simulink model "BMS_V4"  (R2017b)
settings: Solver=FixedStepDiscrete  StartTime=0.0  StopTime=inf  FixedStep=BASETIME  RelTol=1e-3  EnableMultiTasking=on
values from neighbouring files (symbols this model uses):
  AKT_BALANCE = uint16(8)    [BMS_V4_config.m]
  BALANCE = uint16(4)    [BMS_V4_config.m]
  BALANCE_RESISTOR = int32(5)    [BMS_V4_config.m]
  BALANCE_VEC = uint16(8)    [BMS_V4_config.m]
  CELL_SOC = uint16(7)    [BMS_V4_config.m]
  CELL_STATE = uint16(3)    [BMS_V4_config.m]
  CELL_TEMPERATURE = uint16(6)    [BMS_V4_config.m]
  CELL_VOLTAGE = uint16(5)    [BMS_V4_config.m]
  CELLACTBITFIELD = hex2dec('300')    [BMS_V4_config.m]
  CELLDEACTBITFIELD = hex2dec('100')    [BMS_V4_config.m]
  CELLT_BURST = uint16(6)    [BMS_V4_config.m]
  CELLV_BURST = uint16(5)    [BMS_V4_config.m]
  CLK_CYC_timer_1 = 586    [BMS_V4_config.m]
  CLK_CYC_timer_2 = 5860    [BMS_V4_config.m]
  CLK_CYC_timer_3 = 280    [BMS_V4_config.m]
  CLK_CYC_timer_4 = 586*100    (= 58600)    [BMS_V4_config.m]
  CLK_CYC_timer_5 = 5800*2    (= 11600)    [BMS_V4_config.m]
  CLK_CYC_timer_6 = 320    [BMS_V4_config.m]
  CN_CELLS = int32(40*3600)    [BMS_V4_config.m]
  CONTACTOR = uint16(1)    [BMS_V4_config.m]
  CONTACTOR_LOCKED = uint16(0)    [BMS_V4_config.m]
  CONTACTOR_UNLOCKED = uint16(1)    [BMS_V4_config.m]
  DEBUG_SEND_STATES = uint16(hex2dec('01'))    [BMS_V4_config.m]
  DELTA_SOC_BALANCE = int32(5*1e6)    [BMS_V4_config.m]
  DELTA_SOC_BALANCE_OFF = int32(1*1e5)    [BMS_V4_config.m]
  DETERMINE_MODEL_PARAMETER_ACT = uint16(100)    [BMS_V4_config.m]
  DETERMINE_MODEL_PARAMETER_SCC = uint16(101)    [BMS_V4_config.m]
  ERROR = uint16(1)    [BMS_V4_config.m]
  EXTERN_SIGNALS = uint16(1)    [BMS_V4_config.m]
  FREQUENCY_STEPS = uint16([25 50 75 100 150 250 500 750                                      1000 1500 2500 5000 7500                                      10010 10015 10025 10050 10075                                      10100 10150 10250 10500 10750                                      11000 11500])    [BMS_V4_config.m]
  GET_IMAG_PART_MFC = uint16(9)    [BMS_V4_config.m]
  GET_IMAG_PART_MSF = uint16(4)    [BMS_V4_config.m]
  GET_REAL_PART_MFC = uint16(8)    [BMS_V4_config.m]
  GET_REAL_PART_MSF = uint16(3)    [BMS_V4_config.m]
  IMU = uint16(7)    [BMS_V4_config.m]
  IMU_AMP_OFF = uint16(5)    [BMS_V4_config.m]
  IMU_DATA_READ_LOCUS_ACT = uint16(6)    [BMS_V4_config.m]
  IMU_DATA_READ_LOCUS_SCC = uint16(7)    [BMS_V4_config.m]
  IMU_DEBUG = uint16(9)    [BMS_V4_config.m]
  IMU_GET_DATA_MFC = uint16(8)    [BMS_V4_config.m]
  IMU_GET_DATA_MSF = uint16(3)    [BMS_V4_config.m]
  IMU_OFFSET_POLLING = uint16(11)    [BMS_V4_config.m]
  IMU_POLLING = uint16(2)    [BMS_V4_config.m]
  IMU_POWER = uint16(10)    [BMS_V4_config.m]
  IMU_SEND_IMAG = uint16(11)    [BMS_V4_config.m]
  IMU_SEND_REAL = uint16(10)    [BMS_V4_config.m]
  INDEX_IMAGPART = uint16(2)    [BMS_V4_config.m]
  INDEX_REALPART = uint16(1)    [BMS_V4_config.m]
  INFO = uint16(2)    [BMS_V4_config.m]
  INIT_OFFSET_AMPLITUDE = uint16(2)    [BMS_V4_config.m]
  LINE_CURRENT = uint16(3)    [BMS_V4_config.m]
  LINE_CURRENT_CANA = uint16(4)    [BMS_V4_config.m]
  LINE_CURRENT_SWITCH_THRESHOLD = int32(2*1e6)    [BMS_V4_config.m]
  NUM_OF_CELLS = uint16(16)    [BMS_V4_config.m]
  NUM_OF_FREQUENCIES_PSO = uint16(14)    [BMS_V4_config.m]
  NUM_OF_LINES = uint16(1)    [BMS_V4_config.m]
  NUM_OF_PARAMETER = single(5)    [BMS_V4_config.m]
  NUM_OF_SOC_POINTS = uint16(110)    [BMS_V4_config.m]
  P_L_BOUND = single([0.05;0.01;0.1;0.01;0.1])    [BMS_V4_config.m]
  P_U_BOUND = single([0.50;0.20;0.9;0.06;60])    [BMS_V4_config.m]
  PARA_ACT_SEND = uint16(101)    [BMS_V4_config.m]
  PARA_DATA_STORE_ACT = uint16(8)    [BMS_V4_config.m]
  PARA_DATA_STORE_SCC = uint16(9)    [BMS_V4_config.m]
  PARA_SCC_SEND = uint16(102)    [BMS_V4_config.m]
  PARTICLE_INIT = single(create_startparticle(P_L_BOUND,P_U_BOUND,NUM_OF_PARTICLE))    [BMS_V4_config.m]
  POLACT = hex2dec('00000BFF')    [BMS_V4_config.m]
  POLDEACT = hex2dec('000008FF')    [BMS_V4_config.m]
  PSO_PARA_DEBUG = uint16(13)    [BMS_V4_config.m]
  REQUEST_SOC_REF = uint16(1000)    [BMS_V4_config.m]
  SCALE_FACTOR_CH1 = single(0.66666666)    [BMS_V4_config.m]
  SCALE_FACTOR_CH2 = single(0.66666666)    [BMS_V4_config.m]
  SEND_CELL_SOC_ABS = uint16(199)    [BMS_V4_config.m]
  SHUT_DOWN_BALANCE_OFF = uint16(3)    [BMS_V4_config.m]
  SHUT_DOWN_BALANCE_ON = uint16(2)    [BMS_V4_config.m]
  START_IMU_MSL = uint16(3)    [BMS_V4_config.m]
  START_IMU_SCC = uint16(1)    [BMS_V4_config.m]
  SWITCH_IMU_OFF = uint16(2)    [BMS_V4_config.m]
  SWITCH_IMU_ON = uint16(1)    [BMS_V4_config.m]
  SWITCH_IMU_ON_OFF = uint16(4)    [BMS_V4_config.m]
  SYSTEM_DEBUG = uint16(12)    [BMS_V4_config.m]
  TIMEOUT_CANA = uint32(5000)    [BMS_V4_config.m]
  TIMEOUT_GATEWAY = uint32(500)    [BMS_V4_config.m]
  TS_SOC = single(0.010)    [BMS_V4_config.m]
  WARNING = uint16(2)    [BMS_V4_config.m]
libraries: c280xlib x44, c2833xlib x5, simulink x2, c2000lib x1, idelinklib_common x1
(part 7 of 8)

== matlab function BMS_V4/FunctionCall_CANA_RX/handle_imu_debug/proceeding_imu_debug ==
  data: msg input; imu_function data_store_memory; imu_offset data_store_memory; imu_amplitude data_store_memory; START_IMU_MSL parameter; START_IMU_SCC parameter; INIT_OFFSET_AMPLITUDE parameter; user_imu_request data_store_memory; SWITCH_IMU_ON_OFF parameter; imu_CAN_high data_store_memory; imu_CAN_low data_store_memory; SWITCH_IMU_ON parameter; SWITCH_IMU_OFF parameter; imu_on_off data_store_memory; IMU_POWER parameter; IMU parameter; gateway_request data_store_memory
function imu_debug(msg,START_IMU_MSL,START_IMU_SCC,...
    INIT_OFFSET_AMPLITUDE,SWITCH_IMU_ON_OFF, SWITCH_IMU_ON,...
    SWITCH_IMU_OFF, IMU_POWER,IMU)

global imu_function
global imu_offset;
global imu_amplitude;
global user_imu_request;
global imu_CAN_high;
global imu_CAN_low;
global imu_on_off;
global gateway_request;

x1 = uint16(bitand(uint32(hex2dec('000000FF')),bitshift(msg(1),-0)));

if x1 == uint16(START_IMU_SCC)
    %imu_function=START_IMU_SCC;
    user_imu_request=START_IMU_SCC;

    elseif x1 == uint16(INIT_OFFSET_AMPLITUDE) % Offset und Amplitude. 
         imu_offset = uint16(bitand(uint32(hex2dec('0000FFFF')),...
              bitshift(msg(1),-8)));
         imu_amplitude = uint16(bitor(bitand(uint32(hex2dec('000000FF')),...
              bitshift(msg(1),-24)),bitand(uint32(hex2dec('0000FF00')),...
              bitshift(msg(2),8))));
                       
    elseif x1 == START_IMU_MSL %start manual impedance measurement
        user_imu_request=START_IMU_MSL;
        
    elseif x1 == SWITCH_IMU_ON_OFF %start manual impedance measurement
        on_off = uint16(bitand(uint32(hex2dec('000000FF')),bitshift(msg(1),-8)));
        CODE = uint16([IMU_POWER 0 0 0]);
        imu_CAN_high = uint32(0);
        if on_off == SWITCH_IMU_ON %IMU on
           CODE(2) = SWITCH_IMU_ON; %IMU ON  
           imu_on_off = true;
        else
           CODE(2) = SWITCH_IMU_OFF; %IMU OFF   
           imu_on_off = false;

        end
        x1=uint16(bitand(uint16(hex2dec('00ff')),uint16(CODE(1))));
        x2=uint16(bitand(uint16(hex2dec('ff00')),uint16(bitshift(uint16(CODE(2)),8))));
        x3=uint16(bitand(uint16(hex2dec('00ff')),uint16(CODE(3))));
        x4=uint16(bitand(uint16(hex2dec('ff00')),uint16(bitshift(uint16(CODE(4)),8))));
        x11=uint16(bitor(x1,x2));
        x12=uint16(bitor(x3,x4));
        imu_CAN_low=uint32(bitor(uint32(x11),bitshift(uint32(x12),16)));
        gateway_request(IMU) = true;


        
   

else
    
end
end

== matlab function BMS_V4/FunctionCall_timer_2/calculation_soc_CC ==
  data: cell_voltages data_store_memory; TS_SOC parameter; NUM_OF_CELLS parameter; BALANCE_RESISTOR parameter; cell_soc_ABS data_store_memory; cell_soc_CC data_store_memory; CN_CELLS parameter; line_currents data_store_memory; imu_offset_is_set data_store_memory; imu_offset data_store_memory; balance_vector data_store_memory; imu_cc_scc data_store_memory; imu_function data_store_memory; START_IMU_SCC parameter
function calculation_soc_CC(TS_SOC, NUM_OF_CELLS, BALANCE_RESISTOR,CN_CELLS,START_IMU_SCC)

global imu_offset_is_set;
global imu_offset;
global cell_voltages;
global line_currents;
global balance_vector;
global cell_soc_CC;  %SoC cells coulomb counting
global cell_soc_ABS;
global imu_cc_scc;
global imu_function;


% IMU_offset Offsetcurrent in mA!

%dt=TS_SOC*ones(NUM_OF_CELLS,1);

linoNo = uint16(1);

if imu_offset_is_set == true
   Iges=single(...
        (single(balance_vector).* ... % I balance in mA
        (single(cell_voltages)./(single(1e4)*... %voltage in V
        single(BALANCE_RESISTOR))).*single(-1))+... 
        (single(line_currents(linoNo))/single(1e6)));       % line current to A
        Iges=Iges-(single(imu_offset)/single(1e3));
  
else
   Iges=single(...
        (single(balance_vector).* ... % I balance in mA
        (single(cell_voltages)./(single(1e4)*... %voltage in V
        single(BALANCE_RESISTOR))).*single(-1))+... 
        (single(line_currents(linoNo))/single(1e6)));       % line current to A
end
 
if (imu_function == START_IMU_SCC)
    if imu_offset_is_set == true
        Iges_scc = single(line_currents(linoNo))/single(1e6);
        Iges_scc = Iges_scc-(single(imu_offset)/single(1e3));
    else
        Iges_scc = single(line_currents(linoNo))/single(1e6);
    end
    delta_SoC_scc =  int32(((TS_SOC*Iges_scc)/single(CN_CELLS))*1e8);
else
    delta_SoC_scc =  int32(0);
end

Iges_abs = single(line_currents(linoNo))/single(1e6);
delta_SoC_abs =  int32(((TS_SOC*Iges_abs)/single(CN_CELLS))*1e8);

%Coulombcounting
delta_SoC = int32(((TS_SOC*Iges)./single(CN_CELLS))*1e8); % 1% = 1e6 ; 

%10 Ausgabe
%cell_soc_ABS(:,linoNo) = cell_soc_ABS(:,linoNo) + int32(abs(delta_SoC));
cell_soc_ABS = cell_soc_ABS + int32(abs(delta_SoC_abs));
cell_soc_CC(:,linoNo)  = cell_soc_CC(:,linoNo) + delta_SoC;
imu_cc_scc = imu_cc_scc + delta_SoC_scc;

== matlab function BMS_V4/MRAM_control/MRAM_send_command/mram_data_editing ==
  data: mram_address input; data_bytes output; mram_data input
function data_bytes = mram_data_editing(mram_address,mram_data)
% prepare data which should write into MRAM memory

%global mram_address;    %combination of command code and address (uint32)
%global mram_data;       %data to write (uint32)

data_bytes= uint16([0 0 0 0 0 0 0 0]);

if( mram_address == uint32(hex2dec('00'))) 
    %If 0x00 only WREN bit is set
    data_bytes(1) = uint16(6);
else
    data_bytes(1) = uint16(bitand(uint32(255),bitshift(mram_address,-0)));
    data_bytes(2) = uint16(bitand(uint32(255),bitshift(mram_address,-8)));
    data_bytes(3) = uint16(bitand(uint32(255),bitshift(mram_address,-16)));
    data_bytes(4) = uint16(bitand(uint32(255),bitshift(mram_address,-24)));

    data_bytes(5) = uint16(bitand(uint32(255),bitshift(mram_data,-0)));
    data_bytes(6) = uint16(bitand(uint32(255),bitshift(mram_data,-8)));
    data_bytes(7) = uint16(bitand(uint32(255),bitshift(mram_data,-16)));
    data_bytes(8) = uint16(bitand(uint32(255),bitshift(mram_data,-24)));
end

== matlab function BMS_V4/FunctionCall_CANA_RX/handle_system_debug/proceeding_system_debug ==
  data: msg input; SOC_CC_STORE parameter; SOC_ABS_STORE parameter; SOC_CC_READ parameter; SOC_ABS_READ parameter; CHANGE_SOC_CC_VALUE parameter; CHANGE_SOC_ABS_VALUE parameter; cell_soc_CC data_store_memory; cell_soc_ABS data_store_memory; mram_command data_store_memory; READ_SOC_CC_MRAM parameter; READ_SOC_ABS_MRAM parameter; READ_ACT_LOCUS_CELLNO parameter; READ_SCC_LOCUS_CELLNO parameter; mram_cellno_to_read data_store_memory; mram_soc_point_to_read data_store_memory; CHARGE_CELL_WITH_BALANCE_RESISTOR parameter; soc_ref_enable data_store_memory; REQUEST_SOC_REF parameter; MANUAL_SOC_OCV_REF parameter; system_function data_store_memory; RESET_MASTER_SLAVE parameter; SHUT_DOWN_BALANCE_OFF parameter; information_mode data_store_memory; gateway_request data_store_memory; INFO parameter; HARDWARE_RESET parameter; ACTIVATE_BALANCE_CHARGE parameter; DEACTIVATE_BALANCE_CHARGE parameter; BALANCE_CHARGE parameter; IMU_DATA_READ_LOCUS_ACT parameter; IMU_DATA_READ_LOCUS_SCC parameter; user_request_cellno_CANA data_store_memory; user_interface data_store_memory; USER_READ_SCC_FOR_CELLNO parameter; user_request_socpoint_CANA data_store_memory; USER_READ_ACT_FOR_CELLNO parameter; USER_READ_PARA_SCC_FOR_CELLNO parameter; READ_SCC_PARA_CELLNO parameter; READ_ACT_PARA_CELLNO parameter; USER_READ_PARA_ACT_FOR_CELLNO parameter; SET_LAST_SOC_POINT_INDEX parameter; last_soc_point_index data_store_memory; STORE_LAST_SOC_INDEX_SCC parameter; CHANGE_SOC_CC_VALUE_UNBALANCED parameter; NUM_OF_CELLS parameter
function system_debug(msg,SOC_CC_STORE,SOC_ABS_STORE,...
    SOC_CC_READ,SOC_ABS_READ,CHANGE_SOC_CC_VALUE,CHANGE_SOC_ABS_VALUE,...
    READ_SOC_CC_MRAM,READ_SOC_ABS_MRAM,READ_ACT_LOCUS_CELLNO,...
    READ_SCC_LOCUS_CELLNO, CHARGE_CELL_WITH_BALANCE_RESISTOR,...
    REQUEST_SOC_REF, MANUAL_SOC_OCV_REF, RESET_MASTER_SLAVE,...
    SHUT_DOWN_BALANCE_OFF, INFO, HARDWARE_RESET,ACTIVATE_BALANCE_CHARGE,...
    DEACTIVATE_BALANCE_CHARGE,BALANCE_CHARGE, IMU_DATA_READ_LOCUS_ACT,...
IMU_DATA_READ_LOCUS_SCC, USER_READ_SCC_FOR_CELLNO,...
USER_READ_ACT_FOR_CELLNO, USER_READ_PARA_SCC_FOR_CELLNO,...
READ_SCC_PARA_CELLNO, READ_ACT_PARA_CELLNO, USER_READ_PARA_ACT_FOR_CELLNO, SET_LAST_SOC_POINT_INDEX, STORE_LAST_SOC_INDEX_SCC, CHANGE_SOC_CC_VALUE_UNBALANCED, NUM_OF_CELLS)
% System Debug data receive via CAN-A
global cell_soc_CC
global cell_soc_ABS
global mram_command
global mram_cellno_to_read
global mram_soc_point_to_read
global soc_ref_enable;
global system_function;
global user_request_cellno_CANA;
global user_request_socpoint_CANA;
global user_interface;
global last_soc_point_index;
%global information_mode;
%global gateway_request;
%global new_SoC_reference

%decode CAN_message
system_debug_id = uint16(bitand(uint32(hex2dec('FFFF')),...
    bitshift(msg(1),-0)));

% info1 = uint16(bitand(uint32(255),bitshift(msg(1),-8)));
% info2 = uint16(bitand(uint32(255),bitshift(msg(1),-16)));
% info3 = uint16(bitand(uint32(255),bitshift(msg(1),-24)));

switch system_debug_id
    case CHANGE_SOC_CC_VALUE
        value = typecast(msg(2),'int32');
        cell_soc_CC(:,:) = value*int32(1e6);
        mram_command(SOC_CC_STORE)=true;
    case CHANGE_SOC_CC_VALUE_UNBALANCED
        value = typecast(msg(2),'int32');
        cell_soc_CC(:,:) = value*int32(1e6);
        for k=15:1:NUM_OF_CELLS
        cell_soc_CC(k,:) = (value-int32(rand*8))*int32(1e6);
        end
        mram_command(SOC_CC_STORE)=true;
    case CHANGE_SOC_ABS_VALUE
        value = typecast(msg(2),'int32');
        cell_soc_ABS = value*int32(1e6);
        mram_command(SOC_ABS_STORE)=true;
    case READ_SOC_CC_MRAM
        mram_command(SOC_CC_READ)=true;
    %case READ_SOC_ABS_MRAM 
    case READ_SCC_LOCUS_CELLNO
        user_request_cellno_CANA = uint16(bitand(uint32(255),...
            bitshift(msg(2),-0)));
        user_request_socpoint_CANA = uint16(bitand(uint32(255),...
            bitshift(msg(2),-8)));
        user_interface(USER_READ_SCC_FOR_CELLNO) = true;
%         mram_soc_point_to_read  = uint16(bitand(uint32(255),...
%             bitshift(msg(2),-8)));
%         mram_cellno_to_read = uint16(bitand(uint32(255),...
%             bitshift(msg(2),-0)));
%         mram_soc_point_to_read  = uint16(bitand(uint32(255),...
%             bitshift(msg(2),-8)));
%         
%         % if soc_point = 255 then read imu data from last measurement
%         mram_command(IMU_DATA_READ_LOCUS_SCC)=true;
          
    case READ_ACT_LOCUS_CELLNO
        user_request_cellno_CANA = uint16(bitand(uint32(255),...
            bitshift(msg(2),-0)));
        
        user_interface(USER_READ_ACT_FOR_CELLNO) = true;
    
    case READ_ACT_PARA_CELLNO
        user_interface(USER_READ_PARA_ACT_FOR_CELLNO) = true;
        
    case READ_SCC_PARA_CELLNO
        user_request_cellno_CANA = uint16(bitand(uint32(255),...
            bitshift(msg(2),-0)));
        
        user_interface(USER_READ_PARA_SCC_FOR_CELLNO) = true;
        
    case SET_LAST_SOC_POINT_INDEX
        last_soc_point_index = uint16(bitand(uint32(255),...
            bitshift(msg(2),-0)));
        mram_command(STORE_LAST_SOC_INDEX_SCC)=true;
        
    case CHARGE_CELL_WITH_BALANCE_RESISTOR
    
    case MANUAL_SOC_OCV_REF
        system_function(MANUAL_SOC_OCV_REF)=true;
   
    case REQUEST_SOC_REF
        
        if(uint16(bitand(uint32(hex2dec('00FF')),...
            bitshift(msg(1),-16))) > uint16(0))
            soc_ref_enable = true;
        else
            soc_ref_enable = false;
        end
    case RESET_MASTER_SLAVE
        system_function(HARDWARE_RESET)=true;
       % information_mode =  SHUT_DOWN_BALANCE_OFF;
       % gateway_request(INFO) = true;
       
    case ACTIVATE_BALANCE_CHARGE
        system_function(BALANCE_CHARGE)=true;
       % information_mode =  SHUT_DOWN_BALANCE_OFF;
       % gateway_request(INFO) = true;
    case DEACTIVATE_BALANCE_CHARGE
        system_function(BALANCE_CHARGE)=false;
        
       % information_mode =  SHUT_DOWN_BALANCE_OFF;
       % gateway_request(INFO) = true;
       
end

%x5 = uint8(bitand(uint32(255),bitshift(msg(2),-0)));
%x6 = uint8(bitand(uint32(255),bitshift(msg(2),-8)));
%x7 = uint8(bitand(uint32(255),bitshift(msg(2),-16)));
%x8 = uint8(bitand(uint32(255),bitshift(msg(2),-24)));


    
end











% 
% 
% 
% global imu_function
% global imu_offset;
% global imu_amplitude;
% global user_imu_request;
% global imu_CAN_high;
% global imu_CAN_low;
% global imu_on_off;
% global gateway_request;
% 
% x1 = uint16(bitand(uint32(hex2dec('000000FF')),bitshift(msg(1),-0)));
% 
% if x1 == uint16(START_IMU_SCC)
%     imu_function=START_IMU_SCC;
% 
%     elseif x1 == uint16(INIT_OFFSET_AMPLITUDE) % Offset und Amplitude. 
%          imu_offset = uint16(bitand(uint32(hex2dec('0000FFFF')),...
%               bitshift(msg(1),-8)));
%          imu_amplitude = uint16(bitor(bitand(uint32(hex2dec('000000FF')),...
%               bitshift(msg(1),-24)),bitand(uint32(hex2dec('0000FF00')),...
%               bitshift(msg(2),8))));
%                        
%     elseif x1 == START_IMU_MSL %start manual impedance measurement
%         user_imu_request=true;
%         
%     elseif x1 == SWITCH_IMU_ON_OFF %start manual impedance measurement
%         on_off = uint16(bitand(uint32(hex2dec('000000FF')),bitshift(msg(1),-8)));
%         CODE = uint16([IMU_POWER 0 0 0]);
%         imu_CAN_high = uint32(0);
%         if on_off == SWITCH_IMU_ON %IMU on
%            CODE(2) = SWITCH_IMU_ON; %IMU ON  
%            imu_on_off = true;
%         else
%            CODE(2) = SWITCH_IMU_OFF; %IMU OFF   
%            imu_on_off = false;
% 
%         end
%         x1=uint16(bitand(uint16(hex2dec('00ff')),uint16(CODE(1))));
%         x2=uint16(bitand(uint16(hex2dec('ff00')),uint16(bitshift(uint16(CODE(2)),8))));
%         x3=uint16(bitand(uint16(hex2dec('00ff')),uint16(CODE(3))));
%         x4=uint16(bitand(uint16(hex2dec('ff00')),uint16(bitshift(uint16(CODE(4)),8))));
%         x11=uint16(bitor(x1,x2));
%         x12=uint16(bitor(x3,x4));
%         imu_CAN_low=uint32(bitor(uint32(x11),bitshift(uint32(x12),16)));
%         gateway_request(IMU) = true;
% 
% 
%         
%    
% 
% else
%     
% end
% end

== matlab function BMS_V4/FunctionCall_SPI_RX/MATLAB Function ==
  data: rx_data_vector input; y output; spi_rx_msg data_store_memory; mram_value_stored data_store_memory; mram_value_read data_store_memory
function y = fcn(rx_data_vector)
%#codegen
global spi_rx_msg;
global mram_value_stored;
global mram_value_read;

x1=uint16(bitand(uint16(hex2dec('00ff')),uint16(rx_data_vector(5))));
x2=uint16(bitand(uint16(hex2dec('ff00')),...
    uint16(bitshift(uint16(rx_data_vector(6)),8))));
x3=uint16(bitand(uint16(hex2dec('00ff')),...
    uint16(rx_data_vector(7))));
x4=uint16(bitand(uint16(hex2dec('ff00')),...
    uint16(bitshift(uint16(rx_data_vector(8)),8))));

x11=uint16(bitor(x1,x2));
x12=uint16(bitor(x3,x4));

spi_rx_msg = uint32(bitor(uint32(x11),bitshift(uint32(x12),16)));

mram_value_stored = true;
mram_value_read = true;
y = spi_rx_msg;

== stateflow chart BMS_V4/PARAMETER_ESTIMATION_control ==
  state init_parameter_estimation
    en:
  state determine_parameter_scc
    state Init
      en:
      pso_cell_no = uint16(1);
      pso_soc_point = uint16(1);
      //soc_point 1 -101 = 0%-100%
    state load_imu_data_from_mram
      en:
      mram_cellno_to_read = pso_cell_no;
      mram_soc_point_to_read = pso_soc_point;
      mram_command[IMU_DATA_READ_LOCUS_SCC - uint16(1)] = true;
    state prepare_data
      en:
      //ga_determination_reday = false;
      [omega_cell, z_meas_cell] =prepare_data_for_pso_scc();
      //send_ms_uart();
      [p_best_act_cell,best_L2_cell]=particle_swarm_v2(omega_cell,z_meas_cell);
      //send_ms_uart();
    state store_parameter_for_act_cell
      en:
      store_parameter_scc(p_best_act_cell,best_L2_cell,pso_soc_point);
    state store_to_mram
      en:
      para_act_cellno = pso_cell_no;
      mram_command[PARA_DATA_STORE_SCC - uint16(1)] = true;
    state send_parameter
      //send parameter of actual cell
      en:
      para_send_act_cell_CANA = pso_cell_no;
      para_send_act_or_scc_CANA = PARA_SCC_SEND;
      CANA_send_data[PSO_PARA_DEBUG-uint16(1)]=true;
    determine_parameter_scc.Init -> determine_parameter_scc.load_imu_data_from_mram
    (junction 513) -> determine_parameter_scc.load_imu_data_from_mram
    (junction 543) -> (junction 513)
    determine_parameter_scc.load_imu_data_from_mram -> determine_parameter_scc.prepare_data : [mram_command[IMU_DATA_READ_LOCUS_SCC - uint16(1)] == false]
    determine_parameter_scc.prepare_data -> determine_parameter_scc.store_parameter_for_act_cell : //[ga_determination_reday == true]
    determine_parameter_scc.store_parameter_for_act_cell -> (junction 543) [order 1] : //[pso_soc_point < NUM_OF_SOC_POINTS]
        | [pso_soc_point < last_soc_point_index]
        | {pso_soc_point++;}
    (junction 514) -> (junction 543) [order 2]
    determine_parameter_scc.store_parameter_for_act_cell -> store_to_mram [order 2]
    store_to_mram -> determine_parameter_scc.send_parameter : [mram_command[PARA_DATA_STORE_SCC - uint16(1)] == false]
    determine_parameter_scc.send_parameter -> (junction 514) : [CANA_send_data[PSO_PARA_DEBUG-uint16(1)] == false]
        | {pso_cell_no++;
        | pso_soc_point = uint16(1);}
  state determine_parameter_act_and_referenz_soc
    state Init
      en:
      pso_cell_no=uint16(1);
    state load_imu_data_from_mram
      en:
      mram_cellno_to_read = pso_cell_no;
      mram_command[IMU_DATA_READ_LOCUS_ACT - uint16(1)] = true;
    state prepare_data
      en:
      //ga_determination_reday = false;
      [omega_cell, z_meas_cell] =prepare_data_for_pso_act();
      //send_ms_uart();
      [p_best_act_cell,best_L2_cell]=particle_swarm_v2(omega_cell,z_meas_cell);
      //send_ms_uart();
    state store_parameter_for_act_cell
      en:
      store_parameter_act(p_best_act_cell,best_L2_cell);
      para_act_cellno = pso_cell_no;
      mram_command[PARA_DATA_STORE_ACT - uint16(1)] = true;
    state send_parameter
      //send parameter of actual cell
      en:
      para_send_act_cell_CANA = pso_cell_no;
      para_send_act_or_scc_CANA = PARA_ACT_SEND;
      CANA_send_data[PSO_PARA_DEBUG-uint16(1)]=true;
    state read _scc_from_actual_cell [commented out]
    state Referenz_SoC [commented out]
      en:
      reference_soc_from_ga(ga_cell_no);
    determine_parameter_act_and_referenz_soc.Init -> determine_parameter_act_and_referenz_soc.load_imu_data_from_mram
    (junction 484) -> determine_parameter_act_and_referenz_soc.load_imu_data_from_mram
    determine_parameter_act_and_referenz_soc.load_imu_data_from_mram -> determine_parameter_act_and_referenz_soc.prepare_data : [mram_command[IMU_DATA_READ_LOCUS_ACT - uint16(1)] == false]
    (junction 485) -> (junction 484) [order 2]
    determine_parameter_act_and_referenz_soc.prepare_data -> determine_parameter_act_and_referenz_soc.store_parameter_for_act_cell : //[ga_determination_reday == true]
    determine_parameter_act_and_referenz_soc.store_parameter_for_act_cell -> determine_parameter_act_and_referenz_soc.send_parameter : [mram_command[PARA_DATA_STORE_ACT - uint16(1)] == false]
    determine_parameter_act_and_referenz_soc.send_parameter -> (junction 485) : [CANA_send_data[PSO_PARA_DEBUG-uint16(1)] == false]
        | {pso_cell_no++;}
    (default) -> read _scc_from_actual_cell [commented out]
    read _scc_from_actual_cell -> Referenz_SoC [commented out]
  state send_ms_uart [function] [commented out]
  init_parameter_estimation -> determine_parameter_scc.Init [order 2] : [start_pso_scc == true]
      | {pso_determination_ready_scc = false;}
  (junction 514) -> init_parameter_estimation [order 1] : [pso_cell_no > NUM_OF_CELLS]
      | {pso_determination_ready_scc = true;
      | start_pso_scc = false;}
  (junction 485) -> init_parameter_estimation [order 1] : [pso_cell_no > NUM_OF_CELLS]
      | {pso_determination_ready_act = true;
      | start_pso_act = false;}
  init_parameter_estimation -> determine_parameter_act_and_referenz_soc.Init [order 1] : [start_pso_act == true]
      | {pso_determination_ready_act = false;}
  (default) -> init_parameter_estimation
  data: omega function_output single size=[NUM_OF_FREQUENCIES_PSO,1]; z_meas function_output single size=[NUM_OF_FREQUENCIES_PSO,1]; p_set function_input single size=[NUM_OF_PARAMETER,1]; l2_norm function_input single; cell_no function_input uint16; omega function_input single size=[NUM_OF_FREQUENCIES_PSO,1]; Z_meas function_input single size=[NUM_OF_FREQUENCIES_PSO,1]; p_best function_output single size=[NUM_OF_PARAMETER,1] =single([1;1;1;1;1]);; bestL2Norm function_output single; omega function_output single size=[NUM_OF_FREQUENCIES_PSO,1]; z_meas function_output single size=[NUM_OF_FREQUENCIES_PSO,1]; p_set function_input single size=[NUM_OF_PARAMETER,1]; l2_norm function_input single; soc_point function_input double; parameter_one_cell_act data_store_memory; FREQUENCY_STEPS parameter size=[1,NUM_OF_FREQUENCIES]; one_locus_act data_store_memory; omega_cell local single size=[NUM_OF_FREQUENCIES_PSO,1]; z_meas_cell local single size=[NUM_OF_FREQUENCIES_PSO,1]; best_L2_cell local single; p_best_act_cell local single size=[NUM_OF_PARAMETER,1]; pso_cell_no local uint16; NUM_OF_PARAMETER parameter; start_pso_act data_store_memory; PSO_PARA_DEBUG parameter uint16; CANA_send_data data_store_memory; NUM_OF_CELLS parameter; pso_determination_ready_act data_store_memory; determined_soc_ga_alpha data_store_memory; determined_soc_ga_rd data_store_memory; NUM_OF_FREQUENCIES_PSO parameter uint16; P_L_BOUND parameter size=[NUM_OF_PARAMETER,1]; P_U_BOUND parameter size=[NUM_OF_PARAMETER,1]; PARTICLE_INIT parameter size=[NUM_OF_PARAMETER,NUM_OF_PARTICLE]; parameter_one_cell_scc data_store_memory; one_locus_scc data_store_memory; para_send_act_cell_CANA data_store_memory; PARA_SCC_SEND parameter; para_send_act_or_scc_CANA data_store_memory; PARA_ACT_SEND parameter; mram_cellno_to_read data_store_memory; para_act_cellno data_store_memory; mram_command data_store_memory; IMU_DATA_READ_LOCUS_ACT parameter; PARA_DATA_STORE_ACT parameter; pso_determination_ready_scc data_store_memory; start_pso_scc data_store_memory; NUM_OF_SOC_POINTS parameter; mram_soc_point_to_read data_store_memory; pso_soc_point local uint16; IMU_DATA_READ_LOCUS_SCC parameter; PARA_DATA_STORE_SCC parameter; last_soc_point_index data_store_memory
  events: trigger_PARAMETER_ESTIMATION input FUNCTION_CALL_EVENT
  function [omega, z_meas] = prepare_data_for_pso_act:
    | function [omega, z_meas] = prepare_data_for_pso_act()
    | 
    | global one_locus_act;
    | 
    | omega = single(2*pi*(single(FREQUENCY_STEPS(1:14)).*single(1e-3)))';
    | z_meas = single(one_locus_act(1:14,1))+1i*single(one_locus_act(1:14,2));
    | 
    | end
  function store_parameter_act(p_set,l2_norm):
    | function store_parameter_act(p_set,l2_norm)
    | 
    | global parameter_one_cell_act;
    | 
    | parameter_one_cell_act(1:5)=p_set;
    | parameter_one_cell_act(6)=l2_norm;
    | 
    | end
  function reference_soc_from_ga(cell_no):
    | function reference_soc_from_ga(cell_no)
    | 
    | global determined_soc_ga_alpha;
    | global determined_soc_ga_rd;
    | global parameter_set;
    | global parameter_scc;
    | 
    | alpha_x = parameter_set(cell_no,3);
    | rd_x    = parameter_set(cell_no,2);
    | 
    | soc_scc = parameter_scc(:,1);
    | alpha_scc = parameter_scc(:,4);
    | rd_scc = parameter_scc(:,3);
    | 
    | yi_alpha = interp1(alpha_scc,soc_scc,alpha_x,'linear','extrap');
    | yi_rd = interp1(rd_scc,soc_scc,rd_x,'linear','extrap');
    | 
    | value_int32=int32(yi_alpha*1e6);
    | determined_soc_ga_alpha(cell_no) = value_int32; 
    | 
    | value_int32=int32(yi_rd*1e6);
    | determined_soc_ga_rd(cell_no) = value_int32;
    | end
  function [p_best,bestL2Norm]= particle_swarm_v2(omega, Z_meas):
    | function [p_best,bestL2Norm]= particle_swarm_v2(omega, Z_meas)
    | %global pso_determination_reday;
    | %
    | %
    | p_LB = P_L_BOUND;
    | p_UB = P_U_BOUND;
    | startparticle = PARTICLE_INIT;
    | iteration_abbort = single(500);
    | iteration_no = single(1);
    | particle_split = uint16(120);
    | 
    | alpha_max = single(0.9);
    | alpha_min = single(0.2);
    | delta_alpha = (alpha_max - alpha_min)/(iteration_abbort*single(0.5));
    | alpha = alpha_max;
    | a1 = single(1.0);
    | a2 = single(1.3);
    | L2_abbort = single(0.001);
    | chi = single(1);
    | 
    | p_local_best = [startparticle; single(ones(1,length(startparticle)))];
    | v_particle   = single(zeros(5,length(startparticle)));
    | p_global_best = single(ones(6,1));
    | p  = startparticle;
    | 
    | p_global_best_old = p_global_best(6);
    | p_global_best_old2 = p_global_best(6);
    | 
    | abbort_counter = uint16(0);
    | reset_counter = uint16(0);
    | 
    | while((p_global_best(6) > L2_abbort) && (iteration_no < iteration_abbort) && (abbort_counter < uint16(2)))      
    |     if (reset_counter > uint16(30))
    |         reset_counter = uint16(0);
    |         p(:,uint16(1):particle_split)  = startparticle(:,uint16(1):particle_split);
    |         p_local_best(:,uint16(1):particle_split)= [startparticle(:,uint16(1):particle_split); single(ones(uint16(1),particle_split))];
    |         v_particle(:,uint16(1):particle_split) = zeros(uint16(5),particle_split);
    |         p(:,1) = p_global_best(1:5);
    |         if ( ( (p_global_best_old2 - p_global_best(6))/p_global_best_old2) > single(1e-2))      
    |             p_global_best_old2 = p_global_best(6);
    |             abbort_counter = uint16(0);
    |        else
    |             abbort_counter =  abbort_counter + uint16(1);
    |         end        
    |     end
    |      
    |     if ( ((p_global_best_old - p_global_best(6))/p_global_best_old) > single(30e-2))
    |         p_global_best_old =  p_global_best(6);
    |         reset_counter = uint16(0);      
    |     else
    |          reset_counter =  reset_counter + uint16(1);
    |     end
    |     
    |     if(alpha > alpha_min)
    |         alpha = alpha_max-(iteration_no*delta_alpha);
    |     else
    |         alpha = alpha_min; 
    |     end
    |     for ind = uint16(1):uint16(1):uint16(length(startparticle))
    |         Z_func = abs(Z_meas - (p(1,ind) + p(2,ind)./(1i*omega./p(5,ind)+single(1)./...
    |         (single(1)+(p(4,ind).*p(5,ind)./(1i*omega)).^p(3,ind).*sqrt(single(2))))));     
    |         L2_actual =sqrt(sum(Z_func.^2));
    |         if (L2_actual < p_local_best(6,ind))
    |             p_local_best(6,ind)   = L2_actual;
    |             p_local_best(1:5,ind) = p(1:5,ind);
    |         end
    |         if (L2_actual <  p_global_best(6))
    |             p_global_best(6)    = L2_actual;
    |             p_global_best(1:5)  = p(1:5,ind);           
    |         end
    |     end
    |     
    |     for i_particle =  uint16(1):uint16(1):uint16(size(startparticle,2))
    |         for  i_para = uint16(1):uint16(1):uint16(size(startparticle,1))
    |             beta1 = single(rand());
    |             beta2 = single(rand());
    |             v_particle(i_para,i_particle) = chi*(alpha*v_particle(i_para,i_particle)...
    |                 + a1*beta1.*(p_local_best(i_para,i_particle)-p(i_para,i_particle))...
    |                 + a2*beta2.*(p_global_best(i_para)-p(i_para,i_particle)));    
    |                 p(i_para,i_particle) = p(i_para,i_particle) + v_particle(i_para,i_particle);
    |             %limiting according to search space 
    |                 if( p(i_para,i_particle) > p_UB(i_para))
    |                     v_particle(i_para,i_particle) = v_particle(i_para,i_particle)*single((-0.5));
    |                     p(i_para,i_particle) = p_UB(i_para);
    |                 end
    |                 if( p(i_para,i_particle) < p_LB(i_para))
    |                     v_particle(i_para,i_particle) = v_particle(i_para,i_particle)*single((-0.5));
    |                     p(i_para,i_particle) = p_LB(i_para);
    |                 end            
    |         
    |         end % i_para
    |     end % i_particle
    |     iteration_no = iteration_no + single(1);
    | end
    | 
    | bestL2Norm = p_global_best(6);
    | p_best = p_global_best(1:5);
    | 
    | %%
    | %  pso_determination_reday = true;
    | end
  function [omega, z_meas] = prepare_data_for_pso_scc:
    | function [omega, z_meas] = prepare_data_for_pso_scc
    | 
    | global one_locus_scc;
    | 
    | omega = single(2*pi*(single(FREQUENCY_STEPS(1:14)).*single(1e-3)))';
    | z_meas = single(one_locus_scc(1:14,1))+1i*single(one_locus_scc(1:14,2));
    | 
    | end
  function store_parameter_scc(p_set,l2_norm,soc_point):
    | function store_parameter_scc(p_set,l2_norm,soc_point)
    | 
    | global parameter_one_cell_scc;
    | 
    | parameter_one_cell_scc(soc_point,1:5) = p_set;
    | parameter_one_cell_scc(soc_point,6) = l2_norm;
    | 
    | end

== matlab function BMS_V4/FunctionCall_CANA_RX/handle_pso_debug/proceeding_pso_debug ==
  data: msg input; DETERMINE_MODEL_PARAMETER_ACT parameter; start_pso_act data_store_memory; CANA_send_data data_store_memory; DETERMINE_MODEL_PARAMETER_SCC parameter; start_pso_scc data_store_memory
function pso_debug(msg,DETERMINE_MODEL_PARAMETER_ACT,...
DETERMINE_MODEL_PARAMETER_SCC)
% System Debug data receive via CAN-A
global start_pso_act;
global start_pso_scc;
global CANA_send_data; 
%global new_SoC_reference

%decode CAN_message
pso_debug_id = uint16(bitand(uint32(hex2dec('00FF')),...
    bitshift(msg(1),-0)));

% info1 = uint16(bitand(uint32(255),bitshift(msg(1),-8)));
% info2 = uint16(bitand(uint32(255),bitshift(msg(1),-16)));
% info3 = uint16(bitand(uint32(255),bitshift(msg(1),-24)));

switch pso_debug_id
    case DETERMINE_MODEL_PARAMETER_ACT
       start_pso_act=true;
    case DETERMINE_MODEL_PARAMETER_SCC
       start_pso_scc=true;
    case uint16(200)
        CANA_send_data(12)=true;
        
end












% 
% 
% 
% global imu_function
% global imu_offset;
% global imu_amplitude;
% global user_imu_request;
% global imu_CAN_high;
% global imu_CAN_low;
% global imu_on_off;
% global gateway_request;
% 
% x1 = uint16(bitand(uint32(hex2dec('000000FF')),bitshift(msg(1),-0)));
% 
% if x1 == uint16(START_IMU_SCC)
%     imu_function=START_IMU_SCC;
% 
%     elseif x1 == uint16(INIT_OFFSET_AMPLITUDE) % Offset und Amplitude. 
%          imu_offset = uint16(bitand(uint32(hex2dec('0000FFFF')),...
%               bitshift(msg(1),-8)));
%          imu_amplitude = uint16(bitor(bitand(uint32(hex2dec('000000FF')),...
%               bitshift(msg(1),-24)),bitand(uint32(hex2dec('0000FF00')),...
%               bitshift(msg(2),8))));
%                        
%     elseif x1 == START_IMU_MSL %start manual impedance measurement
%         user_imu_request=true;
%         
%     elseif x1 == SWITCH_IMU_ON_OFF %start manual impedance measurement
%         on_off = uint16(bitand(uint32(hex2dec('000000FF')),bitshift(msg(1),-8)));
%         CODE = uint16([IMU_POWER 0 0 0]);
%         imu_CAN_high = uint32(0);
%         if on_off == SWITCH_IMU_ON %IMU on
%            CODE(2) = SWITCH_IMU_ON; %IMU ON  
%            imu_on_off = true;
%         else
%            CODE(2) = SWITCH_IMU_OFF; %IMU OFF   
%            imu_on_off = false;
% 
%         end
%         x1=uint16(bitand(uint16(hex2dec('00ff')),uint16(CODE(1))));
%         x2=uint16(bitand(uint16(hex2dec('ff00')),uint16(bitshift(uint16(CODE(2)),8))));
%         x3=uint16(bitand(uint16(hex2dec('00ff')),uint16(CODE(3))));
%         x4=uint16(bitand(uint16(hex2dec('ff00')),uint16(bitshift(uint16(CODE(4)),8))));
%         x11=uint16(bitor(x1,x2));
%         x12=uint16(bitor(x3,x4));
%         imu_CAN_low=uint32(bitor(uint32(x11),bitshift(uint32(x12),16)));
%         gateway_request(IMU) = true;
% 
% 
%         
%    
% 
% else
%     
% end
% end

== stateflow chart BMS_V4/FunctionCall_limit_monitoring ==
  state limit_monitoring_control [parallel]
    settings: executionOrder=1
    state control
      en:
      [error_state, warning_state] = limit_monitoring();
      du:
      [error_state, warning_state] = limit_monitoring();
    state init_limit_monitoring
      en:
    (default) -> init_limit_monitoring
    init_limit_monitoring -> control : after(TIMER_LIM_MON_STARTUP,sec)
  state error_control [parallel]
    settings: executionOrder=3
    state send_error
      en:
      error_flag = true;
      CANA_send_data[ERROR - uint16(1)] = true;
      system_function[BALANCE_CHARGE-uint16(1)] = false;
    state init_error
      en:
      error_flag = false;
    state error_ready
      en:
    (default) -> init_error
    init_error -> error_ready : after(TIMER_LIM_MON_STARTUP,sec)
    error_ready -> send_error : [error_state[1]>uint16(0)]
  state warning_control [parallel]
    settings: executionOrder=2
    state send_warning
      en:
      CANA_send_data[WARNING - uint16(1)] = true;
    state warning_ready
      en:
    state init_warning
      en:
    (default) -> init_warning
    warning_ready -> send_warning : [warning_state[1] > uint16(0)]
    init_warning -> warning_ready : after(TIMER_LIM_MON_STARTUP,sec)
    send_warning -> warning_ready : [CANA_send_data[WARNING - uint16(1)] == false]
  data: error function_output uint16 size=[1,2]; warning function_output uint16 size=[1,2]; error_flag output boolean size=1; cell_voltages data_store_memory; line_currents data_store_memory; error_state data_store_memory size=1; ERR_V_CELL_HIGH parameter; ERR_V_CELL_LOW parameter; WAR_V_CELL_HIGH parameter; WAR_V_CELL_LOW parameter; ERR_I_BAT_HIGH parameter; ERR_I_BAT_LOW parameter; WAR_I_BAT_HIGH parameter; WAR_I_BAT_LOW parameter; warning_state data_store_memory; ERR_SOC_CELL_HIGH parameter; ERR_SOC_CELL_LOW parameter; WAR_SOC_CELL_HIGH parameter; WAR_SOC_CELL_LOW parameter; CANA_send_data data_store_memory; WARNING parameter; ERROR parameter; TIMER_LIM_MON_STARTUP parameter; ERR_V_BAT_HIGH parameter; ERR_V_BAT_LOW parameter; WAR_V_BAT_HIGH parameter; WAR_V_BAT_LOW parameter; SET_CELL_V_LOW parameter; SET_CELL_V_HIGH parameter; SET_BAT_V_LOW parameter; SET_BAT_V_HIGH parameter; SET_BAT_I_LOW parameter; SET_BAT_I_HIGH parameter; SET_CELL_T_LOW parameter; SET_CELL_T_HIGH parameter; SET_CELL_SOC_LOW parameter; SET_CELL_SOC_HIGH parameter; cell_temperatures data_store_memory; cell_soc_CC data_store_memory; ERR_T_CELL_LOW parameter; WAR_T_CELL_LOW parameter; ERR_T_CELL_HIGH parameter; WAR_T_CELL_HIGH parameter; min_line_current data_store_memory; max_line_current data_store_memory; min_cell_voltage data_store_memory; max_cell_voltage data_store_memory; system_function data_store_memory; balance_vector data_store_memory; BALANCE_CHARGE_V_CELL_MAX parameter; BALANCE_CHARGE parameter; gateway_request data_store_memory; BALANCE parameter; BALANCE_VECTOR_INIT parameter; NUM_OF_CELLS parameter; COUNTER_ERROR parameter
  events: trigger input FUNCTION_CALL_EVENT
  function [error, warning] = limit_monitoring:
    | function [error, warning] = limit_monitoring
    | 
    | global cell_voltages;
    | global line_currents;
    | global cell_temperatures;
    | global cell_soc_CC;
    | global min_cell_voltage;
    | global max_cell_voltage;
    | global min_line_current;
    | global max_line_current;
    | global balance_vector;
    | global system_function;
    | 
    | 
    | persistent warning_flag;
    | persistent warning_check;
    | persistent error_check;
    | 
    | persistent counter_current;
    | 
    | if isempty(counter_current)
    |     counter_current = uint16(1);
    | end
    | 
    | if isempty(warning_flag)
    |     warning_flag = false;
    | end
    | 
    | if isempty(warning_check)
    |     warning_check = uint16([0 0]);
    | end
    | 
    | if isempty(error_check)
    |     error_check = uint16([0 0]);
    | end
    | 
    | 
    | error   = uint16([0 0]);
    | warning = uint16([0 0]);
    | 
    | warning_flag = false;
    | 
    | if(min(cell_voltages) < min_cell_voltage)
    |     min_cell_voltage = min(cell_voltages);
    | end
    | 
    | if(max(cell_voltages) > max_cell_voltage)
    |     max_cell_voltage = max(cell_voltages);
    | end
    | 
    | if(min(line_currents) < min_line_current)
    |    min_line_current = min(line_currents);
    | end
    | 
    | if(max(line_currents) > max_line_current)
    |     max_line_current = max(line_currents);
    | end
    | 
    | 
    | % Cell voltage check min
    | if(min(cell_voltages) < ERR_V_CELL_LOW)
    |     error_check(2) = uint16(1);
    |     error_check(1) = uint16(bitor(error_check(1),SET_CELL_V_LOW));
    | end
    | if (min(cell_voltages) < WAR_V_CELL_LOW)
    |     warning_check(2) = uint16(1);
    |     warning_check(1) = uint16(bitor(warning_check(1),SET_CELL_V_LOW));
    |     warning_flag = true;
    | else
    |     warning_check(1) = uint16(bitand(warning_check(1),bitcmp(SET_CELL_V_LOW)));
    | end
    | 
    | % Cell voltage check max
    | if(max(cell_voltages) > ERR_V_CELL_HIGH)
    |     error_check(2)   = uint16(2);
    |     error_check(1) = uint16(bitor(error_check(1),SET_CELL_V_HIGH));
    | end
    | if (max(cell_voltages) > WAR_V_CELL_HIGH)
    |     warning_check(2) = uint16(2);
    |     warning_check(1) = uint16(bitor(warning_check(1),SET_CELL_V_HIGH));
    |     warning_flag = true;
    | else
    |     warning_check(1) = uint16(bitand(warning_check(1),bitcmp(SET_CELL_V_HIGH)));
    | end
    | 
    | % Battery voltage check min
    | if(sum(uint32(cell_voltages)) < ERR_V_BAT_LOW)
    |     error_check(2) = uint16(3);
    |     error_check(1) = uint16(bitor(error_check(1),SET_BAT_V_LOW));
    | end
    | if (sum(uint32(cell_voltages)) < WAR_V_BAT_LOW)
    |     warning_check(2) = uint16(3);
    |     warning_check(1) = uint16(bitor(warning_check(1),SET_BAT_V_LOW));
    |     warning_flag = true;
    | else
    |     warning_check(1) = uint16(bitand(warning_check(1),bitcmp(SET_BAT_V_LOW)));
    | end
    | 
    | % Battery voltage check max
    | if(sum(uint32(cell_voltages)) > ERR_V_BAT_HIGH)
    |     error_check(2)   = uint16(4);
    |     error_check(1) = uint16(bitor(error_check(1),SET_BAT_V_HIGH));
    | end
    | if (sum(uint32(cell_voltages)) > WAR_V_BAT_HIGH)
    |     warning_check(2) = uint16(4);
    |     warning_check(1) = uint16(bitor(warning_check(1),SET_BAT_V_HIGH));
    |     warning_flag = true;
    | else
    |     warning_check(1) = uint16(bitand(warning_check(1),bitcmp(SET_BAT_V_HIGH)));
    | end
    | 
    | % Current check min
    | if(line_currents < ERR_I_BAT_LOW)
    |     if(counter_current < COUNTER_ERROR)
    |         counter_current = counter_current + uint16(1);
    |     else
    |         error_check(2)   = uint16(5);
    |         error_check(1) = uint16(bitor(error_check(1),SET_BAT_I_LOW));
    |     end
    | else
    |     if(counter_current > uint16(0))
    |         counter_current = uint16(counter_current - uint16(1));
    |     else
    |         counter_current = uint16(0);
    |     end
    | end
    | 
    | if (line_currents < WAR_I_BAT_LOW)
    |     warning_check(2) = uint16(5);
    |     warning_check(1) = uint16(bitor(warning_check(1),SET_BAT_I_LOW));
    |     warning_flag = true;
    | else
    |     warning_check(1) = uint16(bitand(warning_check(1),bitcmp(SET_BAT_I_LOW)));
    | end
    |  
    | % Current check max
    | if(line_currents > ERR_I_BAT_HIGH)
    |     if(counter_current < COUNTER_ERROR)
    |         counter_current = counter_current + uint16(1);
    |     else
    |        error_check(2)   = uint16(6);
    |        error_check(1) = uint16(bitor(error_check(1),SET_BAT_I_HIGH));
    |     end
    | else
    |     if(counter_current > uint16(0))
    |         counter_current = uint16(counter_current - uint16(1));
    |     else
    |         counter_current = uint16(0);
    |     end
    | end
    | 
    | if (line_currents > WAR_I_BAT_HIGH)
    |     warning_check(2) = uint16(6);
    |     warning_check(1) = uint16(bitor(warning_check(1),SET_BAT_I_HIGH));
    |     warning_flag = true;
    | else
    |     warning_check(1) = uint16(bitand(warning_check(1),bitcmp(SET_BAT_I_HIGH)));
    | end
    | 
    | % Cell temperature check min
    | if(min(cell_temperatures) < ERR_T_CELL_LOW)
    |     error_check(2) = uint16(7);
    |     error_check(1) = uint16(bitor(error_check(1),SET_CELL_T_LOW));
    | end
    | if (min(cell_temperatures) < WAR_T_CELL_LOW)
    |     warning_check(2) = uint16(7);
    |     warning_check(1) = uint16(bitor(warning_check(1),SET_CELL_T_LOW));
    |     warning_flag = true;
    | else
    |     warning_check(1) = uint16(bitand(warning_check(1),bitcmp(SET_CELL_T_LOW)));
    | end
    | 
    | % Cell temperature check max
    | if(max(cell_temperatures) > ERR_T_CELL_HIGH)
    |     error_check(2)   = uint16(8);
    |     error_check(1) = uint16(bitor(error_check(1),SET_CELL_T_HIGH));
    | end
    | if (max(cell_temperatures) > WAR_T_CELL_HIGH)
    |     warning_check(2) = uint16(8);
    |     warning_check(1) = uint16(bitor(warning_check(1),SET_CELL_T_HIGH));
    |     warning_flag = true;
    | else
    |     warning_check(1) = uint16(bitand(warning_check(1),bitcmp(SET_CELL_T_HIGH)));
    | end
    | 
    | % Cell soc check min
    | if(min(cell_soc_CC(1)) < ERR_SOC_CELL_LOW)
    |     error_check(2) = uint16(9);
    |     error_check(1) = uint16(bitor(error_check(1),SET_CELL_SOC_LOW));
    | end
    | if (min(cell_soc_CC(1)) < WAR_SOC_CELL_LOW)
    |     warning_check(2) = uint16(9);
    |     warning_check(1) = uint16(bitor(warning_check(1),SET_CELL_SOC_LOW));
    |     warning_flag = true;
    | else
    |     warning_check(1) = uint16(bitand(warning_check(1),bitcmp(SET_CELL_SOC_LOW)));
    | end
    | 
    | % Cell soc check max
    | if(max(cell_soc_CC(1)) > ERR_SOC_CELL_HIGH)
    |     error_check(2)   = uint16(10);
    |     error_check(1) = uint16(bitor(error_check(1),SET_CELL_SOC_HIGH));
    | end
    | if (max(cell_soc_CC(1)) > WAR_SOC_CELL_HIGH)
    |     warning_check(2) = uint16(10);
    |     warning_check(1) = uint16(bitor(warning_check(1),SET_CELL_SOC_HIGH));
    |     warning_flag = true;
    | else
    |     warning_check(1) = uint16(bitand(warning_check(1),bitcmp(SET_CELL_SOC_HIGH)));
    | end
    | 
    | if (warning_flag == false)
    |     warning_check(2) = uint16(0);
    | end
    | 
    | % balance 
    | if (system_function(BALANCE_CHARGE) == true)
    |    line_nr = uint16(1);
    |    for cell_nr = uint16(1):uint16(1):NUM_OF_CELLS
    |        if(cell_voltages(cell_nr,line_nr) > BALANCE_CHARGE_V_CELL_MAX)
    |            balance_vector(cell_nr,line_nr) = true;
    |        end
    | 
    |    end
    |  
    | end
    | 
    | 
    | 
    | error   = error_check;
    | warning = warning_check;
    | end
